simulink model "ex_topmdl_ssreuse"  (R2022b)
settings: configuration reference "Configuration" (kept outside this file)
settings Model: Creator=amyyang  LastModifiedBy=amyyang
settings ConfigSetRef: SourceName=Configuration  SourceLocation=Base Workspace

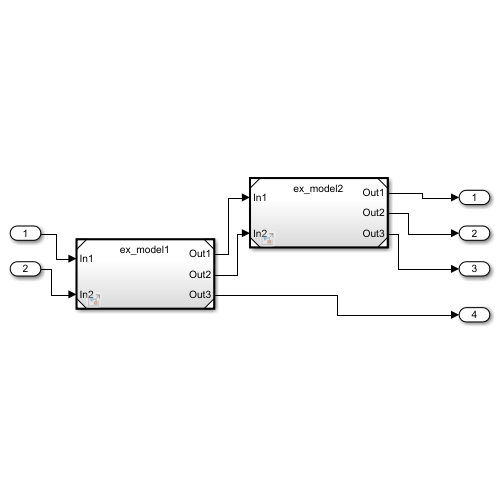
[thumbnail: Simulink's stored preview of the top-level diagram]
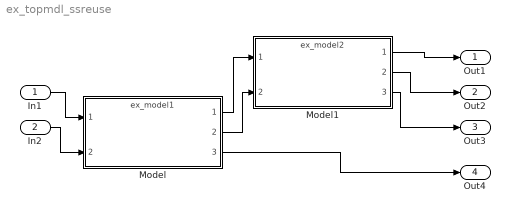
== system ex_topmdl_ssreuse ==
  In1 : Inport
  In2 : Inport  Port=2
  Model : ModelReference  ModelNameDialog=ex_model1.slx  SimulationMode=Normal  ModelReferenceVersion=1.4
  Model1 : ModelReference  ModelNameDialog=ex_model2.slx  SimulationMode=Normal  ModelReferenceVersion=1.8
  Out1 : Outport
  Out2 : Outport  Port=2
  Out3 : Outport  Port=3
  Out4 : Outport  Port=4
  wires:
  Model1/2 -> Out2/1
  In2/1 -> Model/2
  Model1/1 -> Out1/1
  Model/1 -> Model1/1
  In1/1 -> Model/1
  Model/2 -> Model1/2
  Model1/3 -> Out3/1
  Model/3 -> Out4/1
